simulink model "MarchMPC"  (R2023b)
settings: Solver=daessc  StartTime=0.0  StopTime=15  FixedStep=0.01  RelTol=1e-3
values from neighbouring files (symbols this model uses):
  Q = blkdiag(Q, q)    [SolveMPC.m]
undefined symbols (not defined in the file or in its folder): dw_des, LFstates, LRstates, p_cur, p_des, px, py, pz, RFstates, RRstates, v_cur, v_des, vx, vy, vz, w, w_des, X, Y, Z
libraries: sm_lib x57, nesl_utility x47
(part 4 of 4)

== matlab function MarchMPC/Gait/RR ==
  data: t_hip output; t_thigh output; t_shank output; t1 input; t2 input; t3 input; dt1 input; dt2 input; dt3 input; ei input; gait input; ei output; phase input; x0l input; y0l input; z0l input; x0 output; y0 output; z0 output
function [t_hip,t_thigh,t_shank,ei, x0,y0,z0] = leg_controller(t1,t2,t3,dt1,dt2,dt3,ei,gait,phase,x0l,y0l,z0l)
h = 0.3;
T = 0.6;
l1 = 0.2;
l2 = 0.8;
l3 = 0.8;

phase = phase(1);
% xl = q_land(1);
% yl = q_land(2);
% zl = q_land(3);

%% 正运动学部分
if phase <0.0001
    ei = [0;0;0];
    % % x
    x0 = l1*cos(t1) - l3*(sin(t1)*sin(t2)*sin(t3) - cos(t2)*cos(t3)*sin(t1)) + l2*cos(t2)*sin(t1);
    % % y
    y0 = l3*(cos(t1)*sin(t2)*sin(t3) - cos(t1)*cos(t2)*cos(t3)) + l1*sin(t1) - l2*cos(t1)*cos(t2);
    % % z
    z0 = - l3*sin(t2 + t3) - l2*sin(t2);
else
    x0 = x0l;
    y0 = y0l;
    z0 = z0l;
end

flag = gait(1);
switch flag
    case 0
        xl = x0;
        yl = y0;
        zl = z0;
        %% 求解轨迹和速度
        xc = x0 + (xl - x0)/(2*pi)*(2*pi*phase - sin(2*pi*phase));
        zc = z0 + (zl - z0)/(2*pi)*(2*pi*phase - sin(2*pi*phase));
        yc = y0 + h/2*(1 - cos(2*pi*phase))-0.01;

        dxc = (xl - x0)/T*(1 - cos(2*pi*phase));
        dyc = (yl - y0)/T*(1 - cos(2*pi*phase));
        dzc = (pi*h)/T*sin(2*pi*phase);

        %% 逆运动学部分
        % 角度
        L = sqrt(abs(xc^2 + yc^2 - l1^2));
        t1c = atan2((yc * l1 + xc * L),(xc * l1 - yc * L));
        t3c = pi - acos((l2^2 + l3^2 - (xc^2 + yc^2 + zc^2 - l1^2))/(2*l2*l3));
        t2c_t = -(zc + (l3*(yc - (l1*(imag(l1*xc) + real(l1*yc) - imag(yc*(- l1^2 + xc^2 + yc^2)^(1/2)) + real(xc*(- l1^2 + xc^2 + yc^2)^(1/2))))/abs(l1*xc - yc*(- l1^2 + xc^2 + yc^2)^(1/2) + l1*yc*1i + xc*(- l1^2 + xc^2 + yc^2)^(1/2)*1i))*(1 - (l1^2 + l2^2 + l3^2 - xc^2 - yc^2 - zc^2)^2/(4*l2^2*l3^2))^(1/2))/((l2*(imag(l1*yc) - real(l1*xc) + imag(xc*(- l1^2 + xc^2 + yc^2)^(1/2)) + real(yc*(- l1^2 + xc^2 + yc^2)^(1/2))))/abs(l1*xc - yc*(- l1^2 + xc^2 + yc^2)^(1/2) + l1*yc*1i + xc*(- l1^2 + xc^2 + yc^2)^(1/2)*1i) - ((imag(l1*yc) - real(l1*xc) + imag(xc*(- l1^2 + xc^2 + yc^2)^(1/2)) + real(yc*(- l1^2 + xc^2 + yc^2)^(1/2)))*(l1^2 + l2^2 + l3^2 - xc^2 - yc^2 - zc^2))/(2*l2*abs(l1*xc - yc*(- l1^2 + xc^2 + yc^2)^(1/2) + l1*yc*1i + xc*(- l1^2 + xc^2 + yc^2)^(1/2)*1i))))/(l2 - l3*((l1^2 + l2^2 + l3^2 - xc^2 - yc^2 - zc^2)/(2*l2*l3) + (l3*((l1^2 + l2^2 + l3^2 - xc^2 - yc^2 - zc^2)^2/(4*l2^2*l3^2) - 1)*(imag(l1*yc) - real(l1*xc) + imag(xc*(- l1^2 + xc^2 + yc^2)^(1/2)) + real(yc*(- l1^2 + xc^2 + yc^2)^(1/2))))/(abs(l1*xc - yc*(- l1^2 + xc^2 + yc^2)^(1/2) + l1*yc*1i + xc*(- l1^2 + xc^2 + yc^2)^(1/2)*1i)*((l2*(imag(l1*yc) - real(l1*xc) + imag(xc*(- l1^2 + xc^2 + yc^2)^(1/2)) + real(yc*(- l1^2 + xc^2 + yc^2)^(1/2))))/abs(l1*xc - yc*(- l1^2 + xc^2 + yc^2)^(1/2) + l1*yc*1i + xc*(- l1^2 + xc^2 + yc^2)^(1/2)*1i) - ((imag(l1*yc) - real(l1*xc) + imag(xc*(- l1^2 + xc^2 + yc^2)^(1/2)) + real(yc*(- l1^2 + xc^2 + yc^2)^(1/2)))*(l1^2 + l2^2 + l3^2 - xc^2 - yc^2 - zc^2))/(2*l2*abs(l1*xc - yc*(- l1^2 + xc^2 + yc^2)^(1/2) + l1*yc*1i + xc*(- l1^2 + xc^2 + yc^2)^(1/2)*1i))))));
        t2c = asin(t2c_t);

        q_des = [t1c;t2c;t3c];

        % 速度
        J = [l2*cos(t1)*cos(t2) - l1*sin(t1) - l3*(cos(t1)*sin(t2)*sin(t3) - cos(t1)*cos(t2)*cos(t3)), - l3*(cos(t2)*sin(t1)*sin(t3) + cos(t3)*sin(t1)*sin(t2)) - l2*sin(t1)*sin(t2), -l3*(cos(t2)*sin(t1)*sin(t3) + cos(t3)*sin(t1)*sin(t2));
            l1*cos(t1) - l3*(sin(t1)*sin(t2)*sin(t3) - cos(t2)*cos(t3)*sin(t1)) + l2*cos(t2)*sin(t1),   l3*(cos(t1)*cos(t2)*sin(t3) + cos(t1)*cos(t3)*sin(t2)) + l2*cos(t1)*sin(t2),  l3*(cos(t1)*cos(t2)*sin(t3) + cos(t1)*cos(t3)*sin(t2));
            0,                                                - l3*cos(t2 + t3) - l2*cos(t2),                                        -l3*cos(t2 + t3)];
        dq_des_temp = [dxc;dyc;dzc];
        dq_des = J\dq_des_temp;
    case 1
        q_des = [0;0;0];
        dq_des = [0;0;0];
    otherwise
        q_des = [0;0;0];
        dq_des = [0;0;0];
end

q_states = [t1;t2;t3];
dq_states = [dt1;dt2;dt3];

e_q = q_des - q_states;
e_dq = dq_des - dq_states;

%PID参数
kp = [1000;1050;1050];    
ki = [2;2.5;1.5];
kd = [20;85;80];
tqs = kp .* e_q + kd' .* e_dq + ki .* ei; %系统PID控制器输出序列
% Ee = Ee + e_prev;       %累积偏差

t_hip = tqs(1);
t_thigh = tqs(2);
t_shank = tqs(3);
ei = ei + e_q;
end

== matlab function MarchMPC/RobotModeling/RR trqs ==
  data: gait input; t_hip output; strqs input; trqs input; t_thigh output; t_shank output
function [t_hip,t_thigh,t_shank] = choosetrqs(gait,strqs,trqs)
flag = gait(1);
switch flag
    case 0
        t_hip = strqs(1);
        t_thigh = strqs(2);
        t_shank = strqs(3);
    case 1
        t_hip = trqs(1);
        t_thigh = trqs(2);
        t_shank = trqs(3);
    otherwise
        t_hip = 0;
        t_thigh = 0;
        t_shank = 0;
end

== matlab function MarchMPC/RobotModeling/LF trqs ==
  data: gait input; t_hip output; strqs input; trqs input; t_thigh output; t_shank output
function [t_hip,t_thigh,t_shank] = choosetrqs(gait,strqs,trqs)
flag = gait(4);
switch flag
    case 0
        t_hip = strqs(1);
        t_thigh = strqs(2);
        t_shank = strqs(3);
    case 1
        t_hip = trqs(1);
        t_thigh = trqs(2);
        t_shank = trqs(3);
    otherwise
        t_hip = 0;
        t_thigh = 0;
        t_shank = 0;
end

== matlab function MarchMPC/Gait/RF ==
  data: t_hip output; t_thigh output; t_shank output; t1 input; t2 input; t3 input; dt1 input; dt2 input; dt3 input; ei input; gait input; ei output; phase input; x0l input; y0l input; z0l input; x0 output; y0 output; z0 output
function [t_hip,t_thigh,t_shank,ei, x0,y0,z0] = leg_controller(t1,t2,t3,dt1,dt2,dt3,ei,gait,phase,x0l,y0l,z0l)
h = 0.3;
T = 0.6;
l1 = 0.2;
l2 = 0.8;
l3 = 0.8;
phase = phase(2);

% xl = q_land(1);
% yl = q_land(2);
% zl = q_land(3);

%% 正运动学部分
if phase < 0.0001
    ei = [0;0;0];
    % % x
    x0 = l1*cos(t1) - l3*(sin(t1)*sin(t2)*sin(t3) - cos(t2)*cos(t3)*sin(t1)) + l2*cos(t2)*sin(t1);
    % % y
    y0 = l3*(cos(t1)*sin(t2)*sin(t3) - cos(t1)*cos(t2)*cos(t3)) + l1*sin(t1) - l2*cos(t1)*cos(t2);
    % % z
    z0 = - l3*sin(t2 + t3) - l2*sin(t2);
else
    x0 = x0l;
    y0 = y0l;
    z0 = z0l;
end

flag = gait(2);
switch flag
    case 0
        xl = x0;
        yl = y0;
        zl = z0;
        %% 求解轨迹和速度
        xc = x0 + (xl - x0)/(2*pi)*(2*pi*phase - sin(2*pi*phase));
        zc = z0 + (zl - z0)/(2*pi)*(2*pi*phase - sin(2*pi*phase));
        yc = y0 + h/2*(1 - cos(2*pi*phase))-0.01;

        dxc = (xl - x0)/T*(1 - cos(2*pi*phase));
        dyc = (yl - y0)/T*(1 - cos(2*pi*phase));
        dzc = (pi*h)/T*sin(2*pi*phase);

        %% 逆运动学部分
        % 角度
        L = sqrt(abs(xc^2 + yc^2 - l1^2));
        t1c = atan2((yc * l1 + xc * L),(xc * l1 - yc * L));
        t3c = pi - acos((l2^2 + l3^2 - (xc^2 + yc^2 + zc^2 - l1^2))/(2*l2*l3));
        t2c_t = -(zc + (l3*(yc - (l1*(imag(l1*xc) + real(l1*yc) - imag(yc*(- l1^2 + xc^2 + yc^2)^(1/2)) + real(xc*(- l1^2 + xc^2 + yc^2)^(1/2))))/abs(l1*xc - yc*(- l1^2 + xc^2 + yc^2)^(1/2) + l1*yc*1i + xc*(- l1^2 + xc^2 + yc^2)^(1/2)*1i))*(1 - (l1^2 + l2^2 + l3^2 - xc^2 - yc^2 - zc^2)^2/(4*l2^2*l3^2))^(1/2))/((l2*(imag(l1*yc) - real(l1*xc) + imag(xc*(- l1^2 + xc^2 + yc^2)^(1/2)) + real(yc*(- l1^2 + xc^2 + yc^2)^(1/2))))/abs(l1*xc - yc*(- l1^2 + xc^2 + yc^2)^(1/2) + l1*yc*1i + xc*(- l1^2 + xc^2 + yc^2)^(1/2)*1i) - ((imag(l1*yc) - real(l1*xc) + imag(xc*(- l1^2 + xc^2 + yc^2)^(1/2)) + real(yc*(- l1^2 + xc^2 + yc^2)^(1/2)))*(l1^2 + l2^2 + l3^2 - xc^2 - yc^2 - zc^2))/(2*l2*abs(l1*xc - yc*(- l1^2 + xc^2 + yc^2)^(1/2) + l1*yc*1i + xc*(- l1^2 + xc^2 + yc^2)^(1/2)*1i))))/(l2 - l3*((l1^2 + l2^2 + l3^2 - xc^2 - yc^2 - zc^2)/(2*l2*l3) + (l3*((l1^2 + l2^2 + l3^2 - xc^2 - yc^2 - zc^2)^2/(4*l2^2*l3^2) - 1)*(imag(l1*yc) - real(l1*xc) + imag(xc*(- l1^2 + xc^2 + yc^2)^(1/2)) + real(yc*(- l1^2 + xc^2 + yc^2)^(1/2))))/(abs(l1*xc - yc*(- l1^2 + xc^2 + yc^2)^(1/2) + l1*yc*1i + xc*(- l1^2 + xc^2 + yc^2)^(1/2)*1i)*((l2*(imag(l1*yc) - real(l1*xc) + imag(xc*(- l1^2 + xc^2 + yc^2)^(1/2)) + real(yc*(- l1^2 + xc^2 + yc^2)^(1/2))))/abs(l1*xc - yc*(- l1^2 + xc^2 + yc^2)^(1/2) + l1*yc*1i + xc*(- l1^2 + xc^2 + yc^2)^(1/2)*1i) - ((imag(l1*yc) - real(l1*xc) + imag(xc*(- l1^2 + xc^2 + yc^2)^(1/2)) + real(yc*(- l1^2 + xc^2 + yc^2)^(1/2)))*(l1^2 + l2^2 + l3^2 - xc^2 - yc^2 - zc^2))/(2*l2*abs(l1*xc - yc*(- l1^2 + xc^2 + yc^2)^(1/2) + l1*yc*1i + xc*(- l1^2 + xc^2 + yc^2)^(1/2)*1i))))));
        t2c = asin(t2c_t);

        q_des = [t1c;t2c;t3c];

        % 速度
        J = [l2*cos(t1)*cos(t2) - l1*sin(t1) - l3*(cos(t1)*sin(t2)*sin(t3) - cos(t1)*cos(t2)*cos(t3)), - l3*(cos(t2)*sin(t1)*sin(t3) + cos(t3)*sin(t1)*sin(t2)) - l2*sin(t1)*sin(t2), -l3*(cos(t2)*sin(t1)*sin(t3) + cos(t3)*sin(t1)*sin(t2));
            l1*cos(t1) - l3*(sin(t1)*sin(t2)*sin(t3) - cos(t2)*cos(t3)*sin(t1)) + l2*cos(t2)*sin(t1),   l3*(cos(t1)*cos(t2)*sin(t3) + cos(t1)*cos(t3)*sin(t2)) + l2*cos(t1)*sin(t2),  l3*(cos(t1)*cos(t2)*sin(t3) + cos(t1)*cos(t3)*sin(t2));
            0,                                                - l3*cos(t2 + t3) - l2*cos(t2),                                        -l3*cos(t2 + t3)];
        dq_des_temp = [dxc;dyc;dzc];
        dq_des = J\dq_des_temp;
    case 1
        q_des = [0;0;0];
        dq_des = [0;0;0];
    otherwise
        q_des = [0;0;0];
        dq_des = [0;0;0];
end

q_states = [t1;t2;t3];
dq_states = [dt1;dt2;dt3];

e_q = q_des - q_states;
e_dq = dq_des - dq_states;

%PID参数
kp = [1000;1050;1050];    
ki = [2;2.5;1.5];
kd = [20;85;80];
tqs = kp .* e_q + kd' .* e_dq + ki .* ei; %系统PID控制器输出序列
% Ee = Ee + e_prev;       %累积偏差

t_hip = tqs(1);
t_thigh = tqs(2);
t_shank = tqs(3);
ei = ei + e_q;
end

== matlab function MarchMPC/Gait/LF1 ==
  data: t_hip output; t_thigh output; t_shank output; t1 input; t2 input; t3 input; dt1 input; dt2 input; dt3 input; ei input; gait input; ei output; phase input; x0l input; y0l input; z0l input; x0 output; y0 output; z0 output
function [t_hip,t_thigh,t_shank,ei, x0,y0,z0] = leg_controller(t1,t2,t3,dt1,dt2,dt3,ei,gait,phase,x0l,y0l,z0l)
h = 0.3;
T = 0.6;
l1 = 0.2;
l2 = 0.8;
l3 = 0.8;
isRight = -1;
phase = phase(3);

% xl = q_land(1);
% yl = q_land(2);
% zl = q_land(3);

%% 正运动学部分
if phase < 0.0001
    ei = [0;0;0];
    % % x
    x0 = l1*cos(t1) - l3*(sin(t1)*sin(t2)*sin(t3) - cos(t2)*cos(t3)*sin(t1)) + l2*cos(t2)*sin(t1);
    % % y
    y0 = l3*(cos(t1)*sin(t2)*sin(t3) - cos(t1)*cos(t2)*cos(t3)) + l1*sin(t1) - l2*cos(t1)*cos(t2);
    % % z
    z0 = - l3*sin(t2 + t3) - l2*sin(t2);
else
    x0 = x0l;
    y0 = y0l;
    z0 = z0l;
end

flag = gait(3);
switch flag
    case 0
        xl = x0;
        yl = y0;
        zl = z0;
        %% 求解轨迹和速度
        xc = x0 + (xl - x0)/(2*pi)*(2*pi*phase - sin(2*pi*phase));
        zc = z0 + (zl - z0)/(2*pi)*(2*pi*phase - sin(2*pi*phase));
        yc = y0 + h/2*(1 - cos(2*pi*phase))-0.01;

        dxc = (xl - x0)/T*(1 - cos(2*pi*phase));
        dyc = (yl - y0)/T*(1 - cos(2*pi*phase));
        dzc = (pi*h)/T*sin(2*pi*phase);

        %% 逆运动学部分
        % 角度
        L = sqrt(abs(xc^2 + yc^2 - l1^2));
        t1c = atan2((yc * l1 + xc * L),(xc * l1 - yc * L));
        t3c = pi - acos((l2^2 + l3^2 - (xc^2 + yc^2 + zc^2 - l1^2))/(2*l2*l3));
        t2c_t = -(zc + (l3*(yc - (l1*(imag(l1*xc) + real(l1*yc) - imag(yc*(- l1^2 + xc^2 + yc^2)^(1/2)) + real(xc*(- l1^2 + xc^2 + yc^2)^(1/2))))/abs(l1*xc - yc*(- l1^2 + xc^2 + yc^2)^(1/2) + l1*yc*1i + xc*(- l1^2 + xc^2 + yc^2)^(1/2)*1i))*(1 - (l1^2 + l2^2 + l3^2 - xc^2 - yc^2 - zc^2)^2/(4*l2^2*l3^2))^(1/2))/((l2*(imag(l1*yc) - real(l1*xc) + imag(xc*(- l1^2 + xc^2 + yc^2)^(1/2)) + real(yc*(- l1^2 + xc^2 + yc^2)^(1/2))))/abs(l1*xc - yc*(- l1^2 + xc^2 + yc^2)^(1/2) + l1*yc*1i + xc*(- l1^2 + xc^2 + yc^2)^(1/2)*1i) - ((imag(l1*yc) - real(l1*xc) + imag(xc*(- l1^2 + xc^2 + yc^2)^(1/2)) + real(yc*(- l1^2 + xc^2 + yc^2)^(1/2)))*(l1^2 + l2^2 + l3^2 - xc^2 - yc^2 - zc^2))/(2*l2*abs(l1*xc - yc*(- l1^2 + xc^2 + yc^2)^(1/2) + l1*yc*1i + xc*(- l1^2 + xc^2 + yc^2)^(1/2)*1i))))/(l2 - l3*((l1^2 + l2^2 + l3^2 - xc^2 - yc^2 - zc^2)/(2*l2*l3) + (l3*((l1^2 + l2^2 + l3^2 - xc^2 - yc^2 - zc^2)^2/(4*l2^2*l3^2) - 1)*(imag(l1*yc) - real(l1*xc) + imag(xc*(- l1^2 + xc^2 + yc^2)^(1/2)) + real(yc*(- l1^2 + xc^2 + yc^2)^(1/2))))/(abs(l1*xc - yc*(- l1^2 + xc^2 + yc^2)^(1/2) + l1*yc*1i + xc*(- l1^2 + xc^2 + yc^2)^(1/2)*1i)*((l2*(imag(l1*yc) - real(l1*xc) + imag(xc*(- l1^2 + xc^2 + yc^2)^(1/2)) + real(yc*(- l1^2 + xc^2 + yc^2)^(1/2))))/abs(l1*xc - yc*(- l1^2 + xc^2 + yc^2)^(1/2) + l1*yc*1i + xc*(- l1^2 + xc^2 + yc^2)^(1/2)*1i) - ((imag(l1*yc) - real(l1*xc) + imag(xc*(- l1^2 + xc^2 + yc^2)^(1/2)) + real(yc*(- l1^2 + xc^2 + yc^2)^(1/2)))*(l1^2 + l2^2 + l3^2 - xc^2 - yc^2 - zc^2))/(2*l2*abs(l1*xc - yc*(- l1^2 + xc^2 + yc^2)^(1/2) + l1*yc*1i + xc*(- l1^2 + xc^2 + yc^2)^(1/2)*1i))))));
        t2c = asin(t2c_t);

        q_des = isRight * [t1c;t2c;t3c];

        % 速度
        J = [l2*cos(t1)*cos(t2) - l1*sin(t1) - l3*(cos(t1)*sin(t2)*sin(t3) - cos(t1)*cos(t2)*cos(t3)), - l3*(cos(t2)*sin(t1)*sin(t3) + cos(t3)*sin(t1)*sin(t2)) - l2*sin(t1)*sin(t2), -l3*(cos(t2)*sin(t1)*sin(t3) + cos(t3)*sin(t1)*sin(t2));
            l1*cos(t1) - l3*(sin(t1)*sin(t2)*sin(t3) - cos(t2)*cos(t3)*sin(t1)) + l2*cos(t2)*sin(t1),   l3*(cos(t1)*cos(t2)*sin(t3) + cos(t1)*cos(t3)*sin(t2)) + l2*cos(t1)*sin(t2),  l3*(cos(t1)*cos(t2)*sin(t3) + cos(t1)*cos(t3)*sin(t2));
            0,                                                - l3*cos(t2 + t3) - l2*cos(t2),                                        -l3*cos(t2 + t3)];
        dq_des_temp = [dxc;dyc;dzc];
        dq_des = isRight * J\dq_des_temp;
    case 1
        q_des = [0;0;0];
        dq_des = [0;0;0];
    otherwise
        q_des = [0;0;0];
        dq_des = [0;0;0];
end

q_states = [t1;t2;t3];
dq_states = [dt1;dt2;dt3];

e_q = q_des - q_states;
e_dq = dq_des - dq_states;

%PID参数
kp = [1000;1050;1050];    
ki = [2;2.5;1.5];
kd = [20;85;80];
tqs = kp .* e_q + kd' .* e_dq + ki .* ei; %系统PID控制器输出序列
% Ee = Ee + e_prev;       %累积偏差

t_hip = tqs(1);
t_thigh = tqs(2);
t_shank = tqs(3);
ei = ei + e_q;
end

== matlab function MarchMPC/RobotModeling/RF trqs ==
  data: gait input; t_hip output; strqs input; trqs input; t_thigh output; t_shank output
function [t_hip,t_thigh,t_shank] = choosetrqs(gait,strqs,trqs)
flag = gait(2);
switch flag
    case 0
        t_hip = strqs(1);
        t_thigh = strqs(2);
        t_shank = strqs(3);
    case 1
        t_hip = trqs(1);
        t_thigh = trqs(2);
        t_shank = trqs(3);
    otherwise
        t_hip = 0;
        t_thigh = 0;
        t_shank = 0;
end

== matlab function MarchMPC/RobotModeling/LR trqs ==
  data: gait input; t_hip output; strqs input; trqs input; t_thigh output; t_shank output
function [t_hip,t_thigh,t_shank] = choosetrqs(gait,strqs,trqs)
flag = gait(3);
switch flag
    case 0
        t_hip = strqs(1);
        t_thigh = strqs(2);
        t_shank = strqs(3);
    case 1
        t_hip = trqs(1);
        t_thigh = trqs(2);
        t_shank = trqs(3);
    otherwise
        t_hip = 0;
        t_thigh = 0;
        t_shank = 0;
end

== matlab function MarchMPC/Dynamic/RF Converter1 ==
  data: tq1 output size=1; fx input; fy input; fz input; t1 input; t2 input; t3 input; tq2 output size=1; tq3 output size=1
function [tq1,tq2,tq3]= forces2trqs(fx,fy,fz,t1,t2,t3)
Fx = fz;
Fy = fy;
Fz = -fx;
l1 = 0.2;
l2 = 0.8;
l3 = 0.8;
J = [l2*cos(t1)*cos(t2) - l1*sin(t1) - l3*(cos(t1)*sin(t2)*sin(t3) - cos(t1)*cos(t2)*cos(t3)), - l3*(cos(t2)*sin(t1)*sin(t3) + cos(t3)*sin(t1)*sin(t2)) - l2*sin(t1)*sin(t2), -l3*(cos(t2)*sin(t1)*sin(t3) + cos(t3)*sin(t1)*sin(t2));
l1*cos(t1) - l3*(sin(t1)*sin(t2)*sin(t3) - cos(t2)*cos(t3)*sin(t1)) + l2*cos(t2)*sin(t1),   l3*(cos(t1)*cos(t2)*sin(t3) + cos(t1)*cos(t3)*sin(t2)) + l2*cos(t1)*sin(t2),  l3*(cos(t1)*cos(t2)*sin(t3) + cos(t1)*cos(t3)*sin(t2));
                                                                                       0,                                                - l3*cos(t2 + t3) - l2*cos(t2),                                        -l3*cos(t2 + t3)];
tau = -J' * [Fx;Fy;Fz];
tq1 = tau(1);
tq2 = tau(2);
tq3 = tau(3);

== matlab function MarchMPC/Dynamic/RR Converter ==
  data: tq1 output size=1; fx input; fy input; fz input; t1 input; t2 input; t3 input; tq2 output size=1; tq3 output size=1
function [tq1,tq2,tq3]= forces2trqs(fx,fy,fz,t1,t2,t3)

Fx = fz;
Fy = fy;
Fz = -fx;
l1 = 0.2;
l2 = 0.8;
l3 = 0.8;
J = [l2*cos(t1)*cos(t2) - l1*sin(t1) - l3*(cos(t1)*sin(t2)*sin(t3) - cos(t1)*cos(t2)*cos(t3)), - l3*(cos(t2)*sin(t1)*sin(t3) + cos(t3)*sin(t1)*sin(t2)) - l2*sin(t1)*sin(t2), -l3*(cos(t2)*sin(t1)*sin(t3) + cos(t3)*sin(t1)*sin(t2));
l1*cos(t1) - l3*(sin(t1)*sin(t2)*sin(t3) - cos(t2)*cos(t3)*sin(t1)) + l2*cos(t2)*sin(t1),   l3*(cos(t1)*cos(t2)*sin(t3) + cos(t1)*cos(t3)*sin(t2)) + l2*cos(t1)*sin(t2),  l3*(cos(t1)*cos(t2)*sin(t3) + cos(t1)*cos(t3)*sin(t2));
                                                                                       0,                                                - l3*cos(t2 + t3) - l2*cos(t2),                                        -l3*cos(t2 + t3)];
tau = -J' * [Fx;Fy;Fz];
tq1 = tau(1);
tq2 = tau(2);
tq3 = tau(3);

== matlab function MarchMPC/Dynamic/LR Converter2 ==
  data: tq1 output size=1; fx input; fy input; fz input; t1 input; t2 input; t3 input; tq2 output size=1; tq3 output size=1
function [tq1,tq2,tq3]= forces2trqs(fx,fy,fz,t1,t2,t3)
isRight = -1;
Fx = isRight * fz;
Fy = fy;
Fz = -1 * isRight * fx;
l1 = 0.2;
l2 = 0.8;
l3 = 0.8;
J = [l2*cos(t1)*cos(t2) - l1*sin(t1) - l3*(cos(t1)*sin(t2)*sin(t3) - cos(t1)*cos(t2)*cos(t3)), - l3*(cos(t2)*sin(t1)*sin(t3) + cos(t3)*sin(t1)*sin(t2)) - l2*sin(t1)*sin(t2), -l3*(cos(t2)*sin(t1)*sin(t3) + cos(t3)*sin(t1)*sin(t2));
l1*cos(t1) - l3*(sin(t1)*sin(t2)*sin(t3) - cos(t2)*cos(t3)*sin(t1)) + l2*cos(t2)*sin(t1),   l3*(cos(t1)*cos(t2)*sin(t3) + cos(t1)*cos(t3)*sin(t2)) + l2*cos(t1)*sin(t2),  l3*(cos(t1)*cos(t2)*sin(t3) + cos(t1)*cos(t3)*sin(t2));
                                                                                       0,                                                - l3*cos(t2 + t3) - l2*cos(t2),                                        -l3*cos(t2 + t3)];
tau = -J' * [Fx;Fy;Fz];
tq1 = tau(1);
tq2 = tau(2);
tq3 = tau(3);

== matlab function MarchMPC/Dynamic/LF Converter3 ==
  data: tq1 output size=1; fx input; fy input; fz input; t1 input; t2 input; t3 input; tq2 output size=1; tq3 output size=1
function [tq1,tq2,tq3]= forces2trqs(fx,fy,fz,t1,t2,t3)
isRight = -1;
Fx = isRight * fz;
Fy = fy;
Fz = -1 * isRight * fx;
l1 = 0.2;
l2 = 0.8;
l3 = 0.8;
J = [l2*cos(t1)*cos(t2) - l1*sin(t1) - l3*(cos(t1)*sin(t2)*sin(t3) - cos(t1)*cos(t2)*cos(t3)), - l3*(cos(t2)*sin(t1)*sin(t3) + cos(t3)*sin(t1)*sin(t2)) - l2*sin(t1)*sin(t2), -l3*(cos(t2)*sin(t1)*sin(t3) + cos(t3)*sin(t1)*sin(t2));
l1*cos(t1) - l3*(sin(t1)*sin(t2)*sin(t3) - cos(t2)*cos(t3)*sin(t1)) + l2*cos(t2)*sin(t1),   l3*(cos(t1)*cos(t2)*sin(t3) + cos(t1)*cos(t3)*sin(t2)) + l2*cos(t1)*sin(t2),  l3*(cos(t1)*cos(t2)*sin(t3) + cos(t1)*cos(t3)*sin(t2));
                                                                                       0,                                                - l3*cos(t2 + t3) - l2*cos(t2),                                        -l3*cos(t2 + t3)];
tau = -J' * [Fx;Fy;Fz];
tq1 = tau(1);
tq2 = tau(2);
tq3 = tau(3);

== matlab function MarchMPC/MPC-Controller/LegCoorProdunct ==
  data: t1 input; PRRx output; t2 input; t3 input
function PRRx = fcn(t1,t2,t3)
l1 = 0.2;
l2 = 0.8;
l3 = 0.8;

PBRR = [-1.25;0;0.35];
%% 通过正运动学求出足端在腿坐标系中坐标
x = l1*cos(t1) - l3*(sin(t1)*sin(t2)*sin(t3) - cos(t2)*cos(t3)*sin(t1)) + l2*cos(t2)*sin(t1);
y = l3*(cos(t1)*sin(t2)*sin(t3) - cos(t1)*cos(t2)*cos(t3)) + l1*sin(t1) - l2*cos(t1)*cos(t2);
z = - l3*sin(t2 + t3) - l2*sin(t2);

PRR = [-z;y;x];
%% 转换到足端在机体坐标系中的坐标
PTRR = PBRR + PRR;

%% 转换成向量积矩阵
PRRx = [0 -PTRR(3) PTRR(2);
        PTRR(3) 0 -PTRR(1);
        -PTRR(2) PTRR(1) 0];

== matlab function MarchMPC/MPC-Controller/LegCoorProdunct1 ==
  data: t1 input; PRFx output; t2 input; t3 input
function PRFx = fcn(t1,t2,t3)
l1 = 0.2;
l2 = 0.8;
l3 = 0.8;

PBRF = [1.25;0;0.35];
%% 通过正运动学求出足端在腿坐标系中坐标
x = l1*cos(t1) - l3*(sin(t1)*sin(t2)*sin(t3) - cos(t2)*cos(t3)*sin(t1)) + l2*cos(t2)*sin(t1);
y = l3*(cos(t1)*sin(t2)*sin(t3) - cos(t1)*cos(t2)*cos(t3)) + l1*sin(t1) - l2*cos(t1)*cos(t2);
z = - l3*sin(t2 + t3) - l2*sin(t2);

PRF = [-z;y;x];
%% 转换到足端在机体坐标系中的坐标
PTRF = PBRF + PRF;

%% 转换成向量积矩阵
PRFx = [0 -PTRF(3) PTRF(2);
        PTRF(3) 0 -PTRF(1);
        -PTRF(2) PTRF(1) 0];
